simulink model "quad_new_leg_raibert_strategy_v2"  (R2021a)
settings: Solver=ode15s  StartTime=0.0  StopTime=10.0  RelTol=1e-3
undefined symbols (not defined in the file or in its folder): body, ctrl, ground, planner, X, Y, Z
libraries: nesl_utility x73, sm_lib x41, pid_lib x24, simulink x4, Contact_Forces_Lib x4, Parts_Lib x4, sharedtransform x1
(part 5 of 5)

== matlab function quad_new_leg_raibert_strategy_v2/PBC_Dog_Controller/PBC_Core ==
  data: body_pitch input; theta_cmd output; body_pitch_rate input; body_roll input; t input; body_vx input; contact_mux input; leg_fl_state input; leg_fr_state input; leg_rl_state input; leg_rr_state input; pbc_params parameter
function theta_cmd = PBC_Dog_Controller(body_pitch, body_pitch_rate, body_roll, t, body_vx, contact_mux, leg_fl_state, leg_fr_state, leg_rl_state, leg_rr_state, pbc_params)
    % Initialize output vector (16x1)
    theta_cmd = zeros(16, 1);
    pi_val = 3.141592653589793;
    t_d = double(t);

    % --- 1. Parameters Extraction ---
    u_len   = double(pbc_params.upper_length);
    l_len   = double(pbc_params.lower_length);
    stand_h = double(pbc_params.stand_height);
    sw_h    = double(pbc_params.swing_height);
    step_L  = double(pbc_params.step_length);
    T_gait  = double(pbc_params.gait_period);
    duty    = double(pbc_params.duty_factor);

    % --- 2. Mode Management (Smooth State Transition) ---
    % Mode 0: Stand (0-2s), Mode 1: Balance (2-5s), Mode 2: Walk (5s+)
    if t_d < double(pbc_params.stand_time)
        mode = 0; pitch_ref = 90.0; % Start standing up
    elseif t_d < (double(pbc_params.stand_time) + double(pbc_params.balance_time))
        mode = 1; pitch_ref = 90.0; % Hold balance
    else
        mode = 2; pitch_ref = 0.0;  % Start walking
    end

    % --- 3. PBC Potential Energy Shaping (Torque Calculation) ---
    % Calculate Pitch Error (converted to radians)
    e_pitch = (pitch_ref - double(body_pitch)) * (pi_val / 180.0);
    % Damping Injection: We use the rate to "cool down" the system energy
    d_pitch = -double(body_pitch_rate) * (pi_val / 180.0);
    
    % Virtual Spring-Damper Torque (The Core PBC Equation)
    tau_pbc = double(pbc_params.Kp) * sin(e_pitch) + double(pbc_params.Kd) * d_pitch;

    % --- 4. Gait & Phase Synchronization (Trot Gait) ---
    % Leg timing: FL/RR move together, FR/RL move together (180 deg offset)
    phase_fl = mod(t_d / T_gait, 1.0);
    phase_rr = phase_fl;
    phase_fr = mod(t_d / T_gait + 0.5, 1.0);
    phase_rl = phase_fr;

    phases = [phase_fl, phase_fr, phase_rl, phase_rr];
    contacts = [contact_mux(1), contact_mux(2), contact_mux(3), contact_mux(4)];

    % --- 5. Per-Leg Controller Loop ---
    for i = 1:4
        idx = (i-1)*4 + 1;
        p = phases(i);
        swing_dur = 1.0 - duty;

        % Determination of Stance vs Swing
        if mode < 2 || p < duty
            % === STANCE PHASE (Energy Shaping) ===
            % The leg stays at stand_height, but adjusts based on tau_pbc
            % Front legs (i=1,2) and Back legs (i=3,4) respond differently to pitch
            pitch_gain = 0.05; 
            if i > 2, pitch_gain = -0.05; end % Rear legs push opposite to front
            
            target_x = 0.0;
            target_z = stand_h - (tau_pbc * pitch_gain);
        else
            % === SWING PHASE (Cycloidal Trajectory) ===
            % a = normalized swing progress (0 to 1)
            a = (p - duty) / swing_dur;
            if a > 1.0, a = 1.0; end
            
            % X moves smoothly from -HalfStep to +HalfStep
            target_x = step_L * (0.5 - a);
            % Z lifts using a Sine curve (zero velocity at start/end)
            target_z = stand_h - sw_h * sin(pi_val * a);
        end

        % --- 6. Robust Inverse Kinematics (IK) ---
        % Force scalars to prevent dimensionality errors
        [u_cmd, k_cmd] = safe_ik(target_x(1), target_z(1), u_len, l_len);

        theta_cmd(idx)   = 0.0;             % Shoulder (Roll)
        theta_cmd(idx+1) = u_cmd * 180/pi_val; % Upper Leg
        theta_cmd(idx+2) = k_cmd * 180/pi_val; % Knee
        theta_cmd(idx+3) = 1.0;             % Enable Actuator
    end
end

% --- HELPER: Protected Inverse Kinematics ---
function [u, k] = safe_ik(x, z, L1, L2)
    r_sq = x^2 + z^2;
    r = sqrt(r_sq);
    
    % Law of Cosines for Knee (k)
    cos_k = (r_sq - L1^2 - L2^2) / (2 * L1 * L2);
    % Protection: If leg is too short/long, saturate to prevent NaNs
    if cos_k > 1.0, cos_k = 1.0; elseif cos_k < -1.0, cos_k = -1.0; end
    k = acos(cos_k);
    
    % Angle for Upper Leg (u)
    alpha = atan2(z, x);
    cos_u = (r_sq + L1^2 - L2^2) / (2 * r * L1);
    if cos_u > 1.0, cos_u = 1.0; elseif cos_u < -1.0, cos_u = -1.0; end
    u = alpha + acos(cos_u);
end
